simulink model "check_nstm"  (R2018b)
settings: Solver=ode4  StartTime=0.0  StopTime=200  FixedStep=tSPhysics  RelTol=1e-3
libraries: simulink x1
settings Model: DataDictionary=check_nstm.sldd  Creator=wischnewski  LastModifiedBy=ga25xiw
settings DebuggingCC: UnderspecifiedInitializationDetection=Classic  MergeDetectMultiDrivingBlocksExec=none
settings ModelReferenceCC: PropagateSignalLabelsOutOfModel=off

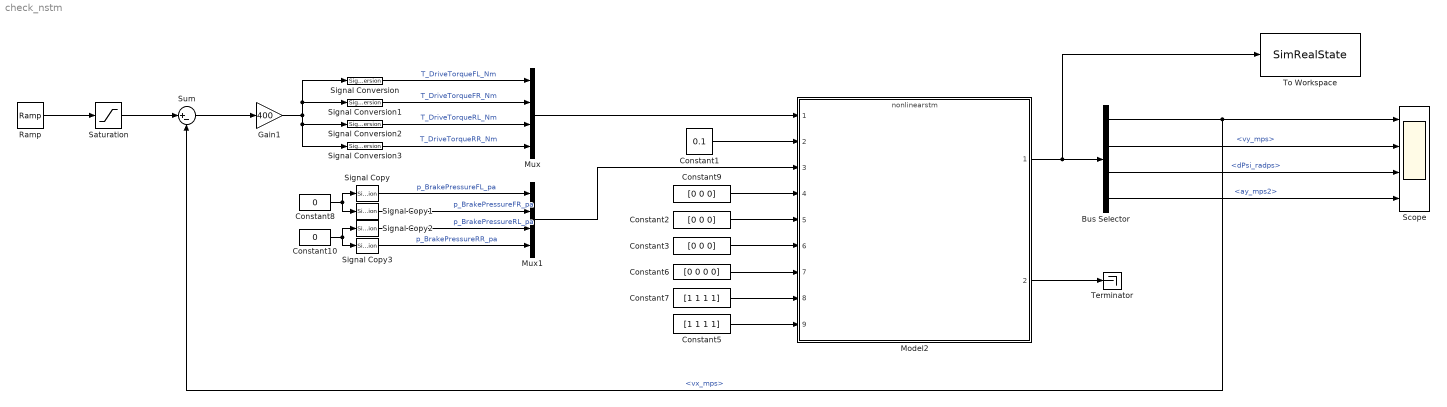
== system check_nstm ==
  Bus Selector : BusSelector  OutputSignals=vx_mps,vy_mps,dPsi_radps,ay_mps2
  Constant1 : Constant  Value=0.1
  Constant10 : Constant  Value=0
  Constant2 : Constant  Value=[0 0 0]
  Constant3 : Constant  Value=[0 0 0]
  Constant5 : Constant  Value=[1 1 1 1]
  Constant6 : Constant  Value=[0 0 0 0]
  Constant7 : Constant  Value=[1 1 1 1]
  Constant8 : Constant  Value=0
  Constant9 : Constant  Value=[0 0 0]
  Gain1 : Gain  Gain=400
  Model2 : ModelReference  ModelNameDialog=nonlinearstm  ParameterArgumentNames=x0_positionstates  ParameterArgumentValues=[0,0,0]  UsingDefaultArgumentValue=0  SimulationMode=Normal  ModelReferenceVersion=1.397
  Mux : Mux
  Mux1 : Mux
  Ramp : simulink/Sources/Ramp  slope=0.15  start=0  InitialOutput=0.1
  Saturation : Saturate  UpperLimit=20  LowerLimit=0
  Scope : Scope  NumInputPorts=4
  Signal Conversion{,1..3} (4 alike) : SignalConversion  OverrideOpt=off
  Signal Copy{,1..3} (4 alike) : SignalConversion  OverrideOpt=off
  Sum : Sum  Inputs=|+-
  Terminator : Terminator
  To Workspace : ToWorkspace  VariableName=SimRealState  SaveFormat=Timeseries  SampleTime=-1
  wires:
  Bus Selector/1 -> Scope/1, Sum/2  "<vx_mps>"
  Bus Selector/2 -> Scope/2  "<vy_mps>"
  Bus Selector/3 -> Scope/3  "<dPsi_radps>"
  Bus Selector/4 -> Scope/4  "<ay_mps2>"
  Model2/1 -> To Workspace/1, Bus Selector/1
  Constant1/1 -> Model2/2
  Signal Conversion/1 -> Mux/1  "T_DriveTorqueFL_Nm"
  Signal Conversion1/1 -> Mux/2  "T_DriveTorqueFR_Nm"
  Signal Conversion2/1 -> Mux/3  "T_DriveTorqueRL_Nm"
  Signal Conversion3/1 -> Mux/4  "T_DriveTorqueRR_Nm"
  Gain1/1 -> Signal Conversion3/1, Signal Conversion2/1, Signal Conversion/1, Signal Conversion1/1
  Sum/1 -> Gain1/1
  Constant9/1 -> Model2/4
  Constant2/1 -> Model2/5
  Constant3/1 -> Model2/6
  Constant6/1 -> Model2/7
  Constant7/1 -> Model2/8
  Constant5/1 -> Model2/9
  Mux/1 -> Model2/1
  Model2/2 -> Terminator/1
  Saturation/1 -> Sum/1
  Ramp/1 -> Saturation/1
  Signal Copy2/1 -> Mux1/3  "p_BrakePressureRL_pa"
  Signal Copy1/1 -> Mux1/2  "p_BrakePressureFR_pa"
  Constant10/1 -> Signal Copy3/1, Signal Copy2/1
  Constant8/1 -> Signal Copy1/1, Signal Copy/1
  Signal Copy/1 -> Mux1/1  "p_BrakePressureFL_pa"
  Signal Copy3/1 -> Mux1/4  "p_BrakePressureRR_pa"
  Mux1/1 -> Model2/3
